simulink model "B00836766_simlulink_lab2"  (R2022b)
settings: Solver=VariableStepAuto  StartTime=0.0  StopTime=4*pi  RelTol=1e-3
libraries: simulink x10
settings Model: Creator=Thomas Wilson  LastModifiedBy=Thomas Wilson

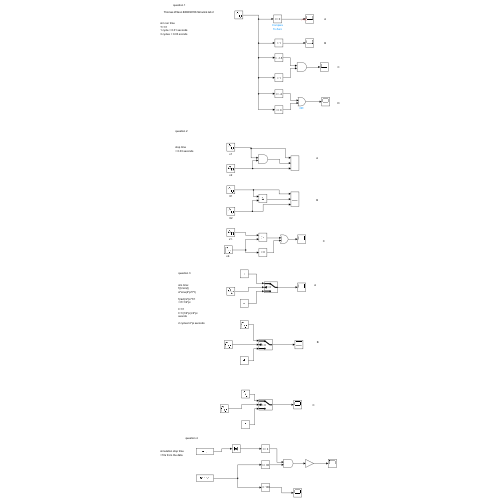
[thumbnail: Simulink's stored preview of the top-level diagram]
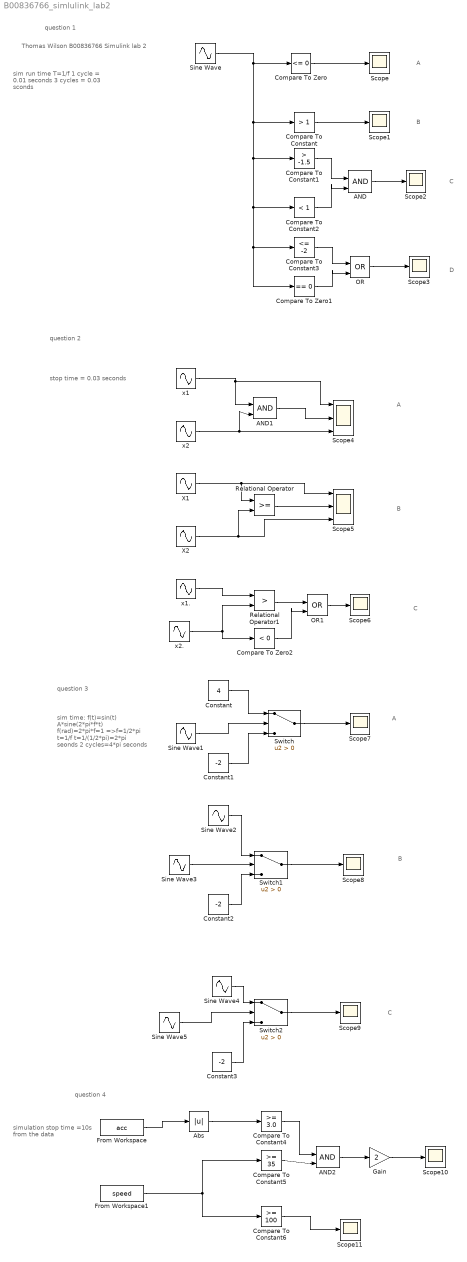
== system B00836766_simlulink_lab2 ==
  note: Thomas Wilson B00836766 Simulink lab 2
  note: sim run time
      | T=1/f
      | 1 cycle = 0.01 seconds
      | 3 cycles = 0.03 sconds
  note: question 1
  note: question 2
  note: A
  note: B
  note: C
  note: D
  note: A
  note: B
  note: C
  note: stop time
      | = 0.03 seconds
  note: question 3
  note: sim time:
      | f(t)=sin(t)
      | A*sine(2*pi*f*t)
      |
      | f(rad)=2*pi*f=1
      | =>f=1/2*pi
      |
      | t=1/f
      | t=1/(1/2*pi)=2*pi
      | seonds
      |
      | 2 cycles=4*pi seconds
  note: A
  note: B
  note: C
  note: question 4
  note: simulation stop time
      | =10s from the data
  AND : Logic  IconShape=distinctive  AllPortsSameDT=off  OutDataTypeStr=boolean
  AND1 : Logic  IconShape=distinctive  AllPortsSameDT=off  OutDataTypeStr=boolean
  AND2 : Logic  IconShape=distinctive  AllPortsSameDT=off  OutDataTypeStr=boolean
  Abs : Abs  SaturateOnIntegerOverflow=off
  Compare To Constant : simulink/Logic and Bit Operations/Compare To Constant  relop=>  const=1  OutDataTypeStr=boolean
  Compare To Constant1 : simulink/Logic and Bit Operations/Compare To Constant  relop=>  const=-1.5  OutDataTypeStr=boolean
  Compare To Constant2 : simulink/Logic and Bit Operations/Compare To Constant  relop=<  const=1  OutDataTypeStr=boolean
  Compare To Constant3 : simulink/Logic and Bit Operations/Compare To Constant  relop=<=  const=-2  OutDataTypeStr=boolean
  Compare To Constant4 : simulink/Logic and Bit Operations/Compare To Constant  relop=>=  const=3.0  OutDataTypeStr=boolean
  Compare To Constant5 : simulink/Logic and Bit Operations/Compare To Constant  relop=>=  const=35  OutDataTypeStr=boolean
  Compare To Constant6 : simulink/Logic and Bit Operations/Compare To Constant  relop=>=  const=100  OutDataTypeStr=boolean
  Compare To Zero : simulink/Logic and Bit Operations/Compare To Zero  relop=<=  OutDataTypeStr=boolean
  Compare To Zero1 : simulink/Logic and Bit Operations/Compare To Zero  relop===  OutDataTypeStr=boolean
  Compare To Zero2 : simulink/Logic and Bit Operations/Compare To Zero  relop=<  OutDataTypeStr=boolean
  Constant : Constant  Value=4
  Constant1 : Constant  Value=-2
  Constant2 : Constant  Value=-2
  Constant3 : Constant  Value=-2
  From Workspace : FromWorkspace  VariableName=acc
  From Workspace1 : FromWorkspace  VariableName=speed
  Gain : Gain  Gain=2
  OR : Logic  Operator=OR  IconShape=distinctive  AllPortsSameDT=off  OutDataTypeStr=boolean
  OR1 : Logic  Operator=OR  IconShape=distinctive  AllPortsSameDT=off  OutDataTypeStr=boolean
  Relational Operator : RelationalOperator  OutDataTypeStr=boolean  RndMeth=Simplest  InputSameDT=off
  Relational Operator1 : RelationalOperator  Operator=>  OutDataTypeStr=boolean  RndMeth=Simplest  InputSameDT=off
  Scope{,1..3,6..11} (10 alike) : Scope
  Scope4 : Scope  NumInputPorts=3
  Scope5 : Scope  NumInputPorts=3
  Sine Wave : Sin  Amplitude=3  Frequency=100*2*pi  SampleTime=0.1e-3
  Sine Wave{1..5} (5 alike) : Sin  SampleTime=0
  Switch : Switch  Criteria=u2 > Threshold  SaturateOnIntegerOverflow=off  InputSameDT=off
  Switch1 : Switch  Criteria=u2 > Threshold  SaturateOnIntegerOverflow=off  InputSameDT=off
  Switch2 : Switch  Criteria=u2 > Threshold  SaturateOnIntegerOverflow=off  InputSameDT=off
  X1 : Sin  Amplitude=5  Frequency=50*2*pi  SampleTime=1/5000
  X2 : Sin  Amplitude=3  Frequency=50*2*pi  SampleTime=1/5000
  x1 : Sin  Amplitude=5  Frequency=50*2*pi  SampleTime=1/5000
  x1. : Sin  Amplitude=5  Frequency=50*2*pi  SampleTime=1/5000
  x2 : Sin  Amplitude=3  Frequency=50*2*pi  SampleTime=1/5000
  x2. : Sin  Amplitude=3  Frequency=50*2*pi  SampleTime=1/5000
  wires:
  ? -> ?
  Sine Wave/1 -> Compare To Zero1/1, Compare To Constant3/1, Compare To Constant2/1, Compare To Constant1/1, Compare To Constant/1, Compare To Zero/1
  Compare To Constant/1 -> Scope1/1
  Compare To Zero/1 -> Scope/1
  Compare To Constant1/1 -> AND/1
  Compare To Constant2/1 -> AND/2
  AND/1 -> Scope2/1
  Compare To Constant3/1 -> OR/1
  Compare To Zero1/1 -> OR/2
  OR/1 -> Scope3/1
  x2/1 -> Scope4/3, AND1/2
  AND1/1 -> Scope4/2
  x1/1 -> Scope4/1, AND1/1
  Relational Operator/1 -> Scope5/2
  X1/1 -> Relational Operator/1, Scope5/1
  X2/1 -> Relational Operator/2, Scope5/3
  x1./1 -> Relational Operator1/1
  OR1/1 -> Scope6/1
  Compare To Zero2/1 -> OR1/2
  Relational Operator1/1 -> OR1/1
  Sine Wave1/1 -> Switch/2
  Constant/1 -> Switch/1
  Constant1/1 -> Switch/3
  Switch/1 -> Scope7/1
  Constant2/1 -> Switch1/3
  Sine Wave2/1 -> Switch1/1
  Sine Wave3/1 -> Switch1/2
  Switch1/1 -> Scope8/1
  Constant3/1 -> Switch2/3
  Sine Wave4/1 -> Switch2/1
  Sine Wave5/1 -> Switch2/2
  Switch2/1 -> Scope9/1
  From Workspace/1 -> Abs/1
  Abs/1 -> Compare To Constant4/1
  Compare To Constant4/1 -> AND2/1
  Compare To Constant5/1 -> AND2/2
  From Workspace1/1 -> Compare To Constant5/1, Compare To Constant6/1
  AND2/1 -> Gain/1
  Gain/1 -> Scope10/1
  Compare To Constant6/1 -> Scope11/1
  x2./1 -> Relational Operator1/2, Compare To Zero2/1
